simulink model "ECCE_tutorial_demo2_part1"  (R2022a)
settings: Solver=FixedStepAuto  StartTime=0.0  StopTime=10/60  FixedStep=1/12000  RelTol=1e-3
undefined symbols (not defined in the file or in its folder): Fault_Inv, GA_th_2, Vdc1, Vdc2, Vdc3, Vdc4, Vdc5
libraries: spsDCVoltageSourceLib x5, spsFullBridgeConverterLib x5, simulink x1, spsSeriesRLCBranchLib x1, spsAlphaBetaZerotodq0Lib x1, spsMeanLib x1, spsVoltageMeasurementLib x1, spspowerguiLib x1
settings Model: Creator=pgm  LastModifiedBy=pgm
settings DataIOCC: ReturnWorkspaceOutputs=off

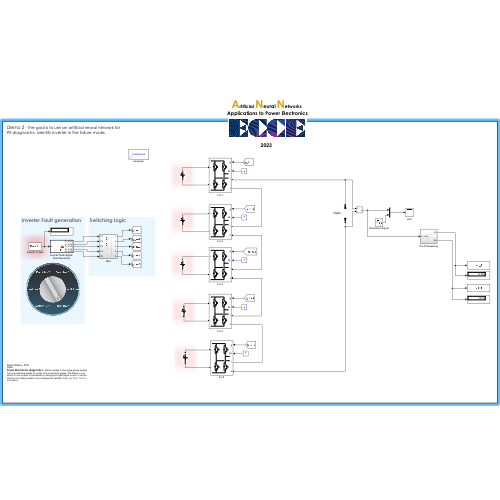
[thumbnail: Simulink's stored preview of the top-level diagram]
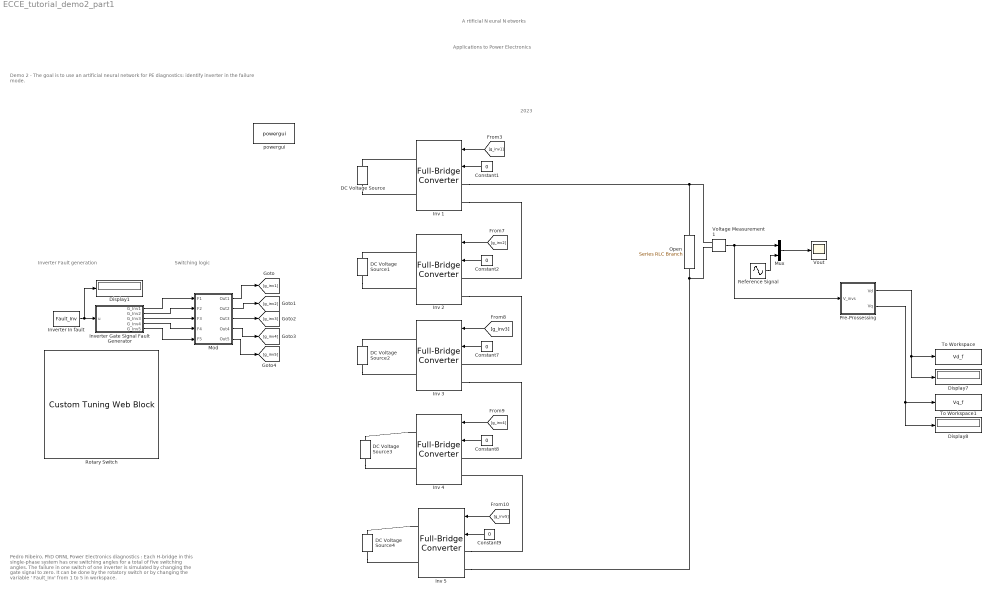
== system ECCE_tutorial_demo2_part1 ==
  note: A rtificial N eural N etworks
  note: Pedro Ribeiro, PhD
      | ORNL
      | Power Electronics diagnostics : Each H-bridge in this single-phase system has one switching angles for a total of five switching angles. The failure in one switch of one inverter is simulated by changing the gate signal to zero. It can be done by the rotatory switch or by changing the variable ' Fault_Inv' from 1 to 5 in workspace.
  note: Applications to Power Electronics
  note: 2023
  note: Demo 2 - The goal is to use an artificial neural network for PE diagnostics: identify inverter in the failure mode.
  note: Switching logic
  note: Inverter Fault generation
  Constant{1..2,7..9} (5 alike) : Constant  Value=0
  DC Voltage Source : spsDCVoltageSourceLib/DC Voltage Source  Amplitude=Vdc1  Measurements=None
  DC Voltage Source1 : spsDCVoltageSourceLib/DC Voltage Source  Amplitude=Vdc2  Measurements=None
  DC Voltage Source2 : spsDCVoltageSourceLib/DC Voltage Source  Amplitude=Vdc3  Measurements=None
  DC Voltage Source3 : spsDCVoltageSourceLib/DC Voltage Source  Amplitude=Vdc4  Measurements=None
  DC Voltage Source4 : spsDCVoltageSourceLib/DC Voltage Source  Amplitude=Vdc5  Measurements=None
  Display1 : Display
  Display7 : Display
  Display8 : Display
  Inv {1..5} (5 alike) : spsFullBridgeConverterLib/Full-Bridge Converter  ModelType=Switching devices  Ron=1e-3  Rs=1e6  Cs=inf  Vforward=[0,0]  Ron_Diode=1e-3  Rs_Diode=1e6  Cs_Diode=inf  Vf_Diode=1e-3  Rs_CurrentSource=inf  Ron_ACsource=1e-3
      settings: SourceProductBaseCode=PS
  Inverter Gate Signal Fault Generator : MATLAB Function  TreatAsAtomicUnit=on
  Inverter In fault : Constant  Value=Fault_Inv
  Mod : Subsystem
  Mux : Mux  Inputs=2
  Open : spsSeriesRLCBranchLib/Series RLC Branch  LConnTagsString=__new0  RConnTagsString=__new0  BranchType=Open circuit  Resistance=50  Inductance=3e-3  SetiL0=off  InitialCurrent=0  Capacitance=400e-6  Setx0=off  InitialVoltage=0  Measurements=None
  Pre-Prossessing : Subsystem
  Reference Signal : Sin  Amplitude=120*sqrt(2)  Frequency=2*pi*60  SampleTime=0
  Rotary Switch : CustomTuningWebBlock  LabelPosition=Hide  ShowInitialText=on  Configuration="{\"components\":[{\"name\":\"RotarySwitchComponent\",\"settings\":{\"arcAngle\":300,\"arcAngleOffset\":120,\"handle\":{\"size\":[150,150],\"src\":\"data:image\\/svg+xml;base64,PHN2ZyBpZD0iTGF5ZXJfMSIgZGF0YS1uYW1lPSJMYXllciAxIiB4bWxucz0iaHR0cDovL3d3dy53My5vcmcvMjAwMC9zdmciIHhtbG5zOnhsaW5rPSJodHRwOi8vd3d3LnczLm9yZy8xOTk5L3hsaW5rIiB2aWV3Qm94PSIwIDAgMTIxIDEyMSI+PGRlZnM+PHN0eWxlPi5jbHMtMXtmaWxsOnVybCgjbGluZWFyLWdyYWRpZW50KTt9LmNscy0yLC5jbHMtM3tmaWxsOiNkMWQxZDE7fS5jbHMtM3tzdHJva2U6I2I3YjdiNztzdHJva2UtbWl0ZXJsaW1pdDoxMDtzdHJva2Utd2lkdGg6MC4yNXB4O30uY2xzLTR7ZmlsbDojZjMwMDAwO30uY2xzLTV7ZmlsbDojZjIxNzY3O308L3N0eWxlPjxsaW5lYXJHcmFkaWVudCBpZD0ibGluZWFyLWdyYWRpZW50IiB4MT0iNjAuNSIgeTE9IjEyMC41IiB4Mj0iNjAuNSIgeTI9IjAuNSIgZ3JhZGllbnRVbml0cz0idXNlclNwYWNlT25Vc2UiPjxzdG9wIG9mZnNldD0iMCIgc3RvcC1jb2xvcj0iI2QxZDFkMSIvPjxzdG9wIG9mZnNldD0iMC4xIiBzdG9wLWNvbG9yPSIjY2VjZWNlIi8+PHN0b3Agb2Zmc2V0PSIwLjE5IiBzdG9wLWNvbG9yPSIjYzNjM2MzIi8+PHN0b3Agb2Zmc2V0PSIwLjI4IiBzdG9wLWNvbG9yPSIjYjFiMWIxIi8+PHN0b3Agb2Zmc2V0PSIwLjM2IiBzdG9wLWNvbG9yPSIjOTg5ODk4Ii8+PHN0b3Agb2Zmc2V0PSIwLjQ0IiBzdG9wLWNvbG9yPSIjNzg3ODc4Ii8+PHN0b3Agb2Zmc2V0PSIwLjQ2IiBzdG9wLWNvbG9yPSIjNmI2YjZiIi8+PHN0b3Agb2Zmc2V0PSIwLjU0IiBzdG9wLWNvbG9yPSIjNmI2YjZiIi8+PHN0b3Agb2Zmc2V0PSIwLjU2IiBzdG9wLWNvbG9yPSIjNzY3Njc2Ii8+PHN0b3Agb2Zmc2V0PSIwLjY0IiBzdG9wLWNvbG9yPSIjOTc5Nzk3Ii8+PHN0b3Agb2Zmc2V0PSIwLjcyIiBzdG9wLWNvbG9yPSIjYjBiMGIwIi8+PHN0b3Agb2Zmc2V0PSIwLjgxIiBzdG9wLWNvbG9yPSIjYzNjM2MzIi8+PHN0b3Agb2Zmc2V0PSIwLjkiIHN0b3AtY29sb3I9IiNjZGNkY2QiLz48c3RvcCBvZmZzZXQ9IjEiIHN0b3AtY29sb3I9IiNkMWQxZDEiLz48L2xpbmVhckdyYWRpZW50PjwvZGVmcz48Y2lyY2xlIGNsYXNzPSJjbHMtMSIgY3g9IjYwLjUiIGN5PSI2MC41IiByPSI2MCIvPjxwYXRoIGNsYXNzPSJjbHMtMiIgZD0iTTYwLjUsMUE1OS41LDU5LjUsMCwxLDEsMSw2MC41LDU5LjU3LDU5LjU3LDAsMCwxLDYwLjUsMW0wLTFBNjAuNSw2MC41LDAsMSwwLDEyMSw2MC41LDYwLjUsNjAuNSwwLDAsMCw2MC41LDBaIi8+PHJlY3QgY2xhc3M9ImNscy0zIiB4PSIwLjUiIHk9IjUxLjUiIHdpZHRoPSIxMjAiIGhlaWdodD0iMTgiIHJ4PSIzLjA0Ii8+PHJlY3QgY2xhc3M9ImNscy00IiB4PSI1Ljc1IiB5PSI1OC43NSIgd2lkdGg9IjE2IiBoZWlnaHQ9IjMiLz48cGF0aCBjbGFzcz0iY2xzLTUiIGQ9Ik0yMS4yNSw1OS4yNXYyaC0xNXYtMmgxNW0xLTFoLTE3djRoMTd2LTRaIi8+PC9zdmc+\"},\"handleOffset\":[0.00839802927552135,0],\"handleOrientation\":180,\"handlePosition\":[0,0,1,1],\"handleSize\":{\"height\":0.5,\"width\":0.5},\"labelRadius\":0.36,\"position\":[0,0,1,1],\"states\":[{\"Label\":{\"color\":[0,0,0,1],\"icon\":{\"size\":[0,0],\"src\":[],\"srcOrientation\":\"Right\"},\"iconPlacement\":\"left\",\"opacity\":1,\"position\":[0.7345552884615385,0.6796274038461538],\"show\":true,\"text\":{\"content\":\"Normal Op.\",\"font\":\"Helvetica\",\"fontSize\":24}},\"Value\":0},{\"Label\":{\"color\":[0,0,0,1],\"icon\":{\"size\":[0,0],\"src\":[],\"srcOrientation\":\"Right\"},\"iconPlacement\":\"left\",\"opacity\":1,\"position\":[0.35757211538461536,0.7603966346153846],\"show\":true,\"text\":{\"content\":\"Fault Inv1\",\"font\":\"Helvetica\",\"fontSize\":24}},\"Value\":1},{\"Label\":{\"color\":[0,0,0,1],\"icon\":{\"size\":[0,0],\"src\":[],\"srcOrientation\":\"Right\"},\"iconPlacement\":\"left\",\"opacity\":1,\"position\":[0.09603365384615385,0.46033653846153844],\"show\":true,\"text\":{\"content\":\"Fault Inv2\",\"font\":\"Helvetica\",\"fontSize\":24}},\"Value\":2},{\"Label\":{\"color\":[0,0,0,1],\"icon\":{\"size\":[0,0],\"src\":[],\"srcOrientation\":\"Right\"},\"iconPlacement\":\"left\",\"opacity\":1,\"position\":[0.36532451923076925,0.1180889423076923],\"show\":true,\"text\":{\"content\":\"Fault Inv3\",\"font\":\"Helvetica\",\"fontSize\":24}},\"Value\":3},{\"Label\":{\"color\":[0,0,0,1],\"icon\":{\"size\":[0,0],\"src\":[],\"srcOrientation\":\"Right\"},\"iconPlacement\":\"left\",\"opacity\":1,\"position\":[0.7191706730769231,0.19501201923076922],\"show\":true,\"text\":{\"content\":\"Fault Inv4\",\"font\":\"Helvetica\",\"fontSize\":24}},\"Value\":4},{\"Label\":{\"color\":[0,0,0],\"icon\":{\"size\":[1,1],\"src\":\"default\",\"srcOrientation\":\"Right\"},\"iconPlacement\":\"left\",\"opacity\":1,\"position\":[0,0],\"show\":true,\"text\":{\"content\":\"Fault Inv5\",\"fontSize\":14}},\"Value\":5}],\"tickRadius\":0.32}},{\"name\":\"BackgroundImageComponent\",\"settings\":{\"image\":{\"size\":[155,150],\"src\":\"data:image\\/svg+xml;base64,PD94bWwgdmVyc2lvbj0iMS4wIiBlbmNvZGluZz0idXRmLTgiPz4NCjwhLS0gR2VuZXJhdG9yOiBBZG9iZSBJbGx1c3RyYXRvciAyNS4wLjAsIFNWRyBFeHBvcnQgUGx1Zy1JbiAuIFNWRyBWZXJzaW9uOiA2LjAwIEJ1aWxkIDApICAtLT4NCjxzdmcgdmVyc2lvbj0iMS4xIg0KCSBpZD0iTGF5ZXJfMl8xXyIgeG1sbnM6Y2M9Imh0dHA6Ly9jcmVhdGl2ZWNvbW1vbnMub3JnL25zIyIgeG1sbnM6ZGM9Imh0dHA6Ly9wdXJsLm9yZy9kYy9lbGVtZW50cy8xLjEvIiB4bWxuczppbmtzY2FwZT0iaHR0cDovL3d3dy5pbmtzY2FwZS5vcmcv ...(+4184 chars)\",\"srcOrientation\":\"Right\"},\"position\":[0,0,1,1],\"scaleMode\":\"0\"}},{\"name\":\"ForegroundImageComponent\",\"settings\":{\"image\":{\"size\":[0,0],\"src\":\"default\",\"srcOrientation\":[]},\"isForeground\":1,\"position\":[0,0,1,1],\"scaleMode\":\"0\"}}],\"settings\":{\"BindingType\":\"param\",\"backgroundColor\":[0,0,255,\"1\"],\"enumDataType\":\"\",\"fixedAspectRatio\":\"on\",\"image\":{\"size\":[150,150],\"src\":\"data:image\\/svg+xml;base64,PD94bWwgdmVyc2lvbj0iMS4wIiBlbmNvZGluZz0iVVRGLTgiIHN0YW5kYWxvbmU9Im5vIj8+CjwhLS0gR2VuZXJhdG9yOiBBZG9iZSBJbGx1c3RyYXRvciAxOS4yLjEsIFNWRyBFeHBvcnQgUGx1Zy1JbiAuIFNWRyBWZXJzaW9uOiA2LjAwIEJ1aWxkIDApICAtLT4KCjxzdmcKICAgeG1sbnM6ZGM9Imh0dHA6Ly9wdXJsLm9yZy9kYy9lbGVtZW50cy8xLjEvIgogICB4bWxuczpjYz0iaHR0cDovL2NyZWF0aXZlY29tbW9ucy5vcmcvbnMjIgogICB4bWxuczpyZGY9Imh0dHA6Ly93d3cudzMub3JnLzE5OTkvMDIvMjItcmRmLXN5bnRh ...(+9660 chars)\"},\"showBackgroundColor\":false,\"useEnumDataType\":false,\"variant\":\"rotarySwitch\"},\"type\":\"RotarySwitch\"}"
  To Workspace : ToWorkspace  VariableName=Vd_f  SampleTime=-1
      settings: MaxDataPoints=1
  To Workspace1 : ToWorkspace  VariableName=Vq_f  SampleTime=-1
      settings: MaxDataPoints=1
  Voltage Measurement1 : spsVoltageMeasurementLib/Voltage Measurement  Tag=PoWeRsYsTeMmEaSuReMeNt  PhasorSimulation=off  OutputType=Magnitude  PSBequivalent=0
  Vout : Scope
  powergui : spspowerguiLib/powergui  Priority=1  SimulationMode=Continuous  SampleTime=1e-6  frequency=60  Iterations=50  frequencyindice=0  Pbase=100e6  ErrMax=1e-4  UnitsV=kV  UnitsW=MW  buscounter=0  FunctionMessages=off  echomessages=off  EnableUseOfTLC=off  CurrentSourceSwitches=off  DisableSnubberDevices=off  DisableRonSwitches=off  DisableVfSwitches=off  DisplayEquations=off  AutomaticDiscreteSolvers=off  SolverType=Tustin/Backward Euler (TBE)  Interpol=off  ExternalGateDelay=off  methode=off  Ts=100  x0status=blocks  SPID=on  SwTol=0  HookPort=off  NonlinearTolerance=1e-4  nMaxIteration=100  ContinueOnMaxIteration=off  RestoreLinks=warning  ResistiveCurrentMeasurement=off  Frange=[0:2:500]  Ylog=off  Xlog=on  ShowGrid=off  save=off  variable=ZData  structure=0  ZoomFFT=off  StartTime=0.0  cycles=1  DisplayStyle=1  fundamental=60  FreqAxis=off  MaxFrequency=1000  frequencyindicesteady=1  RmsSteady=1  display=off
  wires:
  Constant1/1 -> Inv 1/2
  Constant2/1 -> Inv 2/2
  [g_inv1] -> Inv 1/1
  [g_inv2] -> Inv 2/1
  [g_inv4] -> Inv 4/1
  [g_inv3] -> Inv 3/1
  Constant8/1 -> Inv 4/2
  Constant7/1 -> Inv 3/2
  Constant9/1 -> Inv 5/2
  [g_inv5] -> Inv 5/1
  Reference Signal/1 -> Mux/2
  Mux/1 -> Vout/1
  Voltage Measurement1/1 -> Mux/1, Pre-Prossessing/1(V_invs)
  Inverter Gate Signal Fault Generator/1(G_Inv1) -> Mod/1(F1)
  Inverter Gate Signal Fault Generator/2(G_Inv2) -> Mod/2(F2)
  Inverter Gate Signal Fault Generator/3(G_Inv3) -> Mod/3(F3)
  Inverter Gate Signal Fault Generator/4(G_Inv4) -> Mod/4(F4)
  Inverter Gate Signal Fault Generator/5(G_Inv5) -> Mod/5(F5)
  Mod/1(Out1) -> [g_inv1]
  Mod/2(Out2) -> [g_inv2]
  Mod/3(Out3) -> [g_inv3]
  Mod/4(Out4) -> [g_inv4]
  Mod/5(Out5) -> [g_inv5]
  Pre-Prossessing/1(Vd) -> Display7/1, To Workspace/1
  Pre-Prossessing/2(Vq) -> Display8/1, To Workspace1/1
  Inverter In fault/1 -> Display1/1, Inverter Gate Signal Fault Generator/1(u)
  connections:
  DC Voltage Source/RConn1 -- Inv 1/RConn1
  DC Voltage Source/LConn1 -- Inv 1/RConn2
  Inv 2/RConn1 -- DC Voltage Source1/RConn1
  DC Voltage Source1/LConn1 -- Inv 2/RConn2
  Voltage Measurement1/LConn2 -- Inv 5/LConn2 -- Open/RConn1
  Voltage Measurement1/LConn1 -- Inv 1/LConn1 -- Open/LConn1
  Inv 4/RConn1 -- DC Voltage Source3/RConn1
  DC Voltage Source2/LConn1 -- Inv 3/RConn2
  DC Voltage Source3/LConn1 -- Inv 4/RConn2
  DC Voltage Source2/RConn1 -- Inv 3/RConn1
  DC Voltage Source4/LConn1 -- Inv 5/RConn2
  Inv 5/RConn1 -- DC Voltage Source4/RConn1
  Inv 1/LConn2 -- Inv 2/LConn1
  Inv 2/LConn2 -- Inv 3/LConn1
  Inv 3/LConn2 -- Inv 4/LConn1
  Inv 5/LConn1 -- Inv 4/LConn2

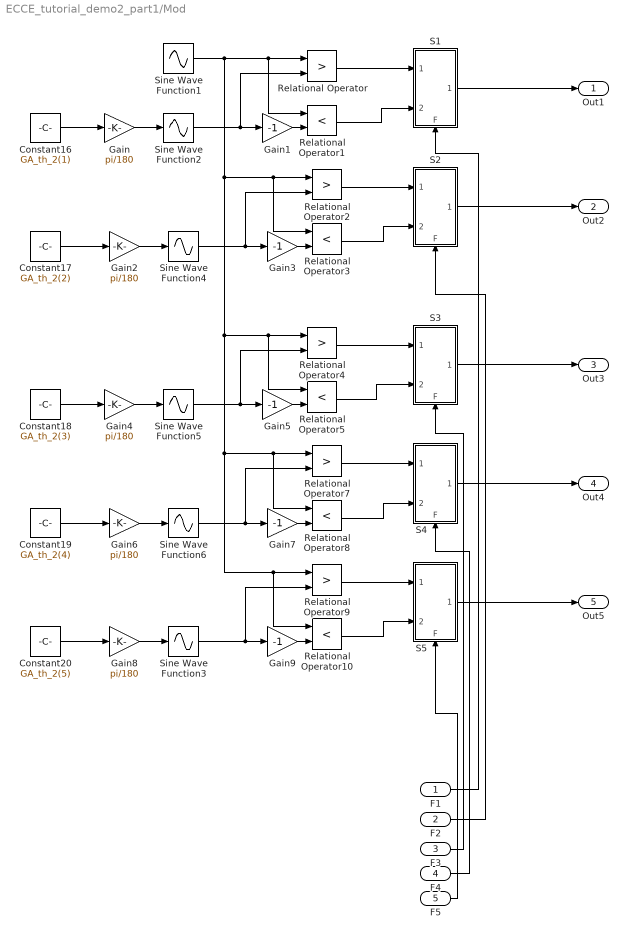
== system ECCE_tutorial_demo2_part1/Mod ==
  F1 : Inport
  F2 : Inport  Port=2
  F3 : Inport  Port=3
  F4 : Inport  Port=4
  F5 : Inport  Port=5
  Constant16 : Constant  Value=GA_th_2(1)
  Constant17 : Constant  Value=GA_th_2(2)
  Constant18 : Constant  Value=GA_th_2(3)
  Constant19 : Constant  Value=GA_th_2(4)
  Constant20 : Constant  Value=GA_th_2(5)
  Gain{,2,4,6,8} (5 alike) : Gain  Gain=pi/180
  Gain{1,3,5,7,9} (5 alike) : Gain  Gain=-1
  Relational Operator{,2,4,7,9} (5 alike) : RelationalOperator  Operator=>  OutDataTypeStr=boolean  RndMeth=Simplest  InputSameDT=off
  Relational Operator{1,3,5,8,10} (5 alike) : RelationalOperator  Operator=<  OutDataTypeStr=boolean  RndMeth=Simplest  InputSameDT=off
  S1 : Subsystem
      settings: PortSchema="{\"entries\":[{\"content\":{\"sides\":[{\"content\":{\"connectorIds\":[\"In1\",\"In2\"]},\"type\":\"ConnectorPlacement.EquallySpacedRectSide\",\"uuid\":\"5f14345d-2d5d-483d-90d8-8aa8f8d7da25\"},{\"content\":{\"connectorIds\":[\"Out1\"],\"side\":\"RIGHT\"},\"type\":\"ConnectorPlacement.EquallySpacedRectSide\",\"uuid\":\"3e161696-ca31-43e2-b7bf-a13ac7fb6ba1\"},{\"content\":{\"connectorIds\":[],\"side\":\"TOP\"},\"type\":\"ConnectorPlacement.EquallySpacedRectSide\",\"uuid\":\"8fa02895-2f1e-47bd-8a65-8e37c65d1a87\"},{\"content\":{\"connectorIds\":[\"In3\"],\"side\":\"BOTTOM\"},\"type\":\"ConnectorPlacement.EquallySpacedRectSide\",\"uuid\":\"36cd283d-056f-45a3-b6f0-6bf0daee5395\"}]},\"type\":\"ConnectorPlacement.EquallySpacedConnector\",\"uuid\":\"d0616103-6a76-4dfd-bdc2-221e478031b1\"}],\"packageUris\":[\"http://schema.mathworks.com/mf0/Connector/R2020b\"],\"version\":\"1.0\"}"
  S2 : Subsystem
      settings: PortSchema="{\"entries\":[{\"content\":{\"sides\":[{\"content\":{\"connectorIds\":[\"In1\",\"In2\"]},\"type\":\"ConnectorPlacement.EquallySpacedRectSide\",\"uuid\":\"5f14345d-2d5d-483d-90d8-8aa8f8d7da25\"},{\"content\":{\"connectorIds\":[\"Out1\"],\"side\":\"RIGHT\"},\"type\":\"ConnectorPlacement.EquallySpacedRectSide\",\"uuid\":\"3e161696-ca31-43e2-b7bf-a13ac7fb6ba1\"},{\"content\":{\"connectorIds\":[],\"side\":\"TOP\"},\"type\":\"ConnectorPlacement.EquallySpacedRectSide\",\"uuid\":\"8fa02895-2f1e-47bd-8a65-8e37c65d1a87\"},{\"content\":{\"connectorIds\":[\"In3\"],\"side\":\"BOTTOM\"},\"type\":\"ConnectorPlacement.EquallySpacedRectSide\",\"uuid\":\"712a4502-34e9-4038-bdd0-4ff6e3ff4ab9\"}]},\"type\":\"ConnectorPlacement.EquallySpacedConnector\",\"uuid\":\"d0616103-6a76-4dfd-bdc2-221e478031b1\"}],\"packageUris\":[\"http://schema.mathworks.com/mf0/Connector/R2020b\"],\"version\":\"1.0\"}"
  S3 : Subsystem
      settings: PortSchema="{\"entries\":[{\"content\":{\"sides\":[{\"content\":{\"connectorIds\":[\"In1\",\"In2\"]},\"type\":\"ConnectorPlacement.EquallySpacedRectSide\",\"uuid\":\"5f14345d-2d5d-483d-90d8-8aa8f8d7da25\"},{\"content\":{\"connectorIds\":[\"Out1\"],\"side\":\"RIGHT\"},\"type\":\"ConnectorPlacement.EquallySpacedRectSide\",\"uuid\":\"3e161696-ca31-43e2-b7bf-a13ac7fb6ba1\"},{\"content\":{\"connectorIds\":[],\"side\":\"TOP\"},\"type\":\"ConnectorPlacement.EquallySpacedRectSide\",\"uuid\":\"8fa02895-2f1e-47bd-8a65-8e37c65d1a87\"},{\"content\":{\"connectorIds\":[\"In3\"],\"side\":\"BOTTOM\"},\"type\":\"ConnectorPlacement.EquallySpacedRectSide\",\"uuid\":\"dcf360f9-50cf-4544-a649-25291c772c87\"}]},\"type\":\"ConnectorPlacement.EquallySpacedConnector\",\"uuid\":\"d0616103-6a76-4dfd-bdc2-221e478031b1\"}],\"packageUris\":[\"http://schema.mathworks.com/mf0/Connector/R2020b\"],\"version\":\"1.0\"}"
  S4 : Subsystem
      settings: PortSchema="{\"entries\":[{\"content\":{\"sides\":[{\"content\":{\"connectorIds\":[\"In1\",\"In2\"]},\"type\":\"ConnectorPlacement.EquallySpacedRectSide\",\"uuid\":\"5f14345d-2d5d-483d-90d8-8aa8f8d7da25\"},{\"content\":{\"connectorIds\":[\"Out1\"],\"side\":\"RIGHT\"},\"type\":\"ConnectorPlacement.EquallySpacedRectSide\",\"uuid\":\"3e161696-ca31-43e2-b7bf-a13ac7fb6ba1\"},{\"content\":{\"connectorIds\":[],\"side\":\"TOP\"},\"type\":\"ConnectorPlacement.EquallySpacedRectSide\",\"uuid\":\"8fa02895-2f1e-47bd-8a65-8e37c65d1a87\"},{\"content\":{\"connectorIds\":[\"In3\"],\"side\":\"BOTTOM\"},\"type\":\"ConnectorPlacement.EquallySpacedRectSide\",\"uuid\":\"86d75a55-3df2-435d-b886-235f200f3608\"}]},\"type\":\"ConnectorPlacement.EquallySpacedConnector\",\"uuid\":\"d0616103-6a76-4dfd-bdc2-221e478031b1\"}],\"packageUris\":[\"http://schema.mathworks.com/mf0/Connector/R2020b\"],\"version\":\"1.0\"}"
  S5 : Subsystem
      settings: PortSchema="{\"entries\":[{\"content\":{\"sides\":[{\"content\":{\"connectorIds\":[\"In1\",\"In2\"]},\"type\":\"ConnectorPlacement.EquallySpacedRectSide\",\"uuid\":\"5f14345d-2d5d-483d-90d8-8aa8f8d7da25\"},{\"content\":{\"connectorIds\":[\"Out1\"],\"side\":\"RIGHT\"},\"type\":\"ConnectorPlacement.EquallySpacedRectSide\",\"uuid\":\"3e161696-ca31-43e2-b7bf-a13ac7fb6ba1\"},{\"content\":{\"connectorIds\":[],\"side\":\"TOP\"},\"type\":\"ConnectorPlacement.EquallySpacedRectSide\",\"uuid\":\"8fa02895-2f1e-47bd-8a65-8e37c65d1a87\"},{\"content\":{\"connectorIds\":[\"In3\"],\"side\":\"BOTTOM\"},\"type\":\"ConnectorPlacement.EquallySpacedRectSide\",\"uuid\":\"319f308e-a951-488d-98cf-79dcc4f9ddf4\"}]},\"type\":\"ConnectorPlacement.EquallySpacedConnector\",\"uuid\":\"d0616103-6a76-4dfd-bdc2-221e478031b1\"}],\"packageUris\":[\"http://schema.mathworks.com/mf0/Connector/R2020b\"],\"version\":\"1.0\"}"
  Sine Wave Function1 : Sin  Frequency=2*pi*60  SampleTime=0
  Sine Wave Function{2..6} (5 alike) : Sin  TimeSource=Use external signal  SampleTime=0
  Out1 : Outport
  Out2 : Outport  Port=2
  Out3 : Outport  Port=3
  Out4 : Outport  Port=4
  Out5 : Outport  Port=5
  wires:
  Gain5/1 -> Relational Operator5/2
  Relational Operator10/1 -> S5/2(In1)
  Relational Operator4/1 -> S3/1(In2)
  Sine Wave Function2/1 -> Gain1/1, Relational Operator/2
  Sine Wave Function3/1 -> Relational Operator9/2, Gain9/1
  Gain4/1 -> Sine Wave Function5/1
  Relational Operator/1 -> S1/1(In2)
  Sine Wave Function4/1 -> Relational Operator2/2, Gain3/1
  Relational Operator9/1 -> S5/1(In2)
  Gain9/1 -> Relational Operator10/2
  S5/1(Out1) -> Out5/1
  Gain/1 -> Sine Wave Function2/1
  Sine Wave Function1/1 -> Relational Operator4/1, Relational Operator5/1, Relational Operator9/1, Relational Operator10/1, Relational Operator8/1, Relational Operator7/1, Relational Operator2/1, Relational Operator3/1, Relational Operator1/1, Relational Operator/1
  Gain7/1 -> Relational Operator8/2
  Gain6/1 -> Sine Wave Function6/1
  Sine Wave Function6/1 -> Gain7/1, Relational Operator7/2
  Sine Wave Function5/1 -> Relational Operator4/2, Gain5/1
  S2/1(Out1) -> Out2/1
  Relational Operator3/1 -> S2/2(In1)
  Constant20/1 -> Gain8/1
  S3/1(Out1) -> Out3/1
  F2/1 -> S2/3(F)
  F1/1 -> S1/3(F)
  Relational Operator2/1 -> S2/1(In2)
  Relational Operator1/1 -> S1/2(In1)
  Constant17/1 -> Gain2/1
  Constant16/1 -> Gain/1
  Gain3/1 -> Relational Operator3/2
  Relational Operator8/1 -> S4/2(In1)
  Gain1/1 -> Relational Operator1/2
  Gain2/1 -> Sine Wave Function4/1
  Constant19/1 -> Gain6/1
  Relational Operator7/1 -> S4/1(In2)
  Constant18/1 -> Gain4/1
  Relational Operator5/1 -> S3/2(In1)
  Gain8/1 -> Sine Wave Function3/1
  S1/1(Out1) -> Out1/1
  S4/1(Out1) -> Out4/1
  F4/1 -> S4/3(F)
  F5/1 -> S5/3(F)
  F3/1 -> S3/3(F)

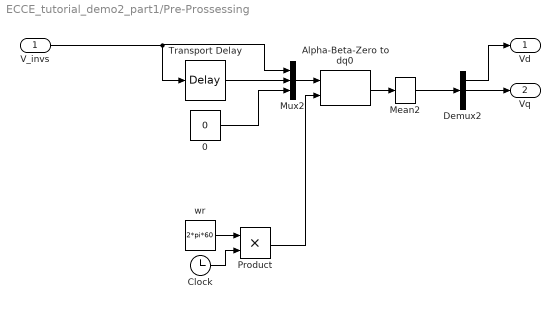
== system ECCE_tutorial_demo2_part1/Pre-Prossessing ==
  V_invs : Inport
  0 : Constant  Value=0
  Alpha-Beta-Zero to dq0 : spsAlphaBetaZerotodq0Lib/Alpha-Beta-Zero to dq0  Alignment=Aligned with phase A axis
      settings: SourceProductBaseCode=PS
  Clock : Clock
  Demux2 : Demux  Outputs=3
  Mean2 : spsMeanLib/Mean  Freq=60  Vinit=0  Ts=0
  Mux2 : Mux  Inputs=3
  Product : Product
  Transport Delay : TransportDelay  DelayTime=(1/60)/4
  wr : Constant  Value=2*pi*60
  Vd : Outport
  Vq : Outport  Port=2
  wires:
  Mux2/1 -> Alpha-Beta-Zero to dq0/1
  Mean2/1 -> Demux2/1
  Demux2/2 -> Vq/1
  Product/1 -> Alpha-Beta-Zero to dq0/2
  Transport Delay/1 -> Mux2/2
  wr/1 -> Product/1
  Clock/1 -> Product/2
  0/1 -> Mux2/3
  Alpha-Beta-Zero to dq0/1 -> Mean2/1
  V_invs/1 -> Mux2/1, Transport Delay/1
  Demux2/1 -> Vd/1

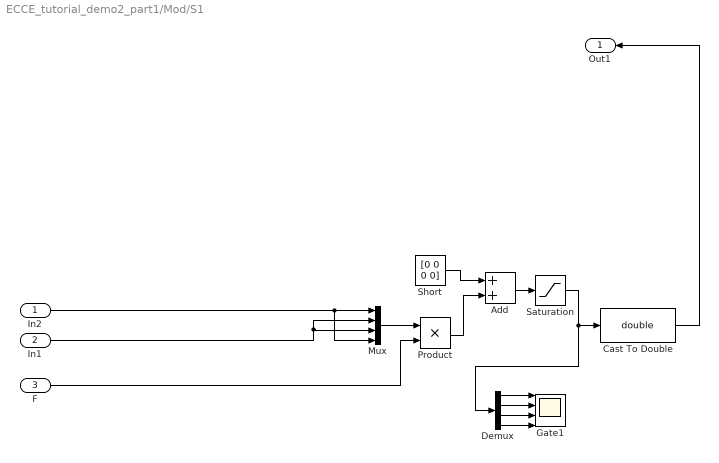
== system ECCE_tutorial_demo2_part1/Mod/S1 ==
  In2 : Inport
  In1 : Inport  Port=2
  F : Inport  Port=3
  Add : Sum
  Cast To Double : DataTypeConversion  OutDataTypeStr=double  SaturateOnIntegerOverflow=off  RndMeth=Floor
  Demux : Demux
  Gate1 : Scope  NumInputPorts=4
  Mux : Mux
  Product : Product
  Saturation : Saturate  UpperLimit=1  LowerLimit=0
  Short : Constant  Value=[0 0 0 0]
  Out1 : Outport
  wires:
  Mux/1 -> Product/1
  Cast To Double/1 -> Out1/1
  In2/1 -> Mux/4, Mux/1
  In1/1 -> Mux/3, Mux/2
  Product/1 -> Add/2
  Demux/1 -> Gate1/1
  Demux/2 -> Gate1/2
  Demux/3 -> Gate1/3
  Demux/4 -> Gate1/4
  Short/1 -> Add/1
  Add/1 -> Saturation/1
  Saturation/1 -> Demux/1, Cast To Double/1
  F/1 -> Product/2

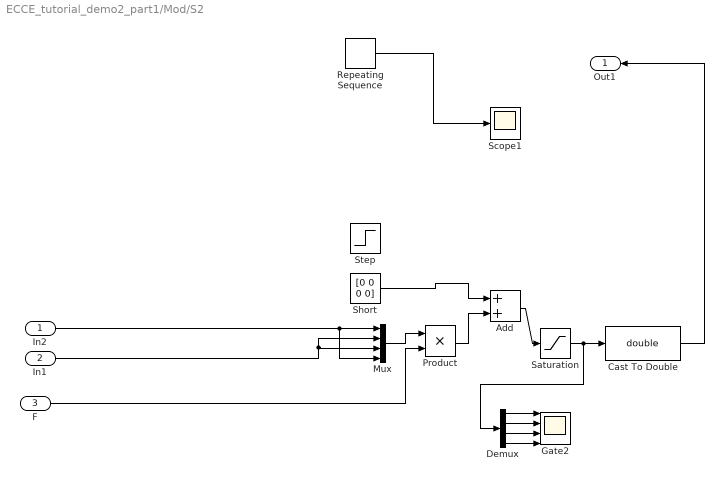
== system ECCE_tutorial_demo2_part1/Mod/S2 ==
  In2 : Inport
  In1 : Inport  Port=2
  F : Inport  Port=3
  Add : Sum
  Cast To Double : DataTypeConversion  OutDataTypeStr=double  SaturateOnIntegerOverflow=off  RndMeth=Floor
  Demux : Demux
  Gate2 : Scope  NumInputPorts=4
  Mux : Mux
  Product : Product
  Repeating Sequence : simulink/Sources/Repeating Sequence  rep_seq_t="[0  3/60 3.01/60 20/60 20.01/60 30/60 ]"  rep_seq_y="[1 1  1 1 1 1 ]"
  Saturation : Saturate  UpperLimit=1  LowerLimit=0
  Scope1 : Scope
  Short : Constant  Value=[0 0 0 0]
  Step : Step  Time=10/60  SampleTime=0
  Out1 : Outport
  wires:
  Repeating Sequence/1 -> Scope1/1
  Short/1 -> Add/1
  Saturation/1 -> Cast To Double/1, Demux/1
  Add/1 -> Saturation/1
  Demux/4 -> Gate2/4
  Demux/3 -> Gate2/3
  Demux/2 -> Gate2/2
  Demux/1 -> Gate2/1
  Product/1 -> Add/2
  In1/1 -> Mux/2, Mux/3
  In2/1 -> Mux/1, Mux/4
  Cast To Double/1 -> Out1/1
  Mux/1 -> Product/1
  F/1 -> Product/2

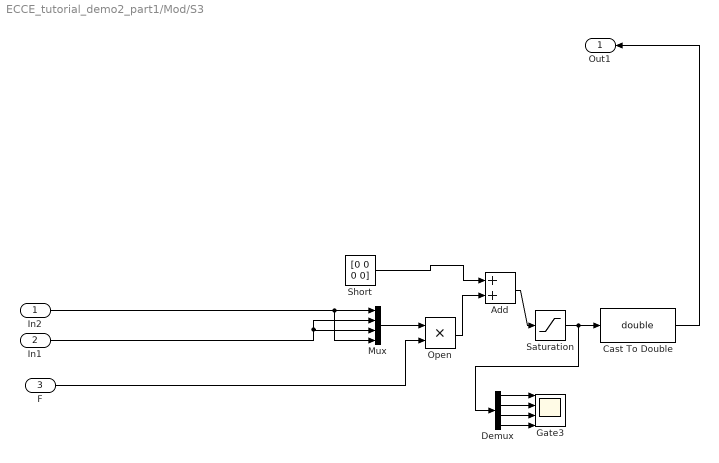
== system ECCE_tutorial_demo2_part1/Mod/S3 ==
  In2 : Inport
  In1 : Inport  Port=2
  F : Inport  Port=3
  Add : Sum
  Cast To Double : DataTypeConversion  OutDataTypeStr=double  SaturateOnIntegerOverflow=off  RndMeth=Floor
  Demux : Demux
  Gate3 : Scope  NumInputPorts=4
  Mux : Mux
  Open : Product
  Saturation : Saturate  UpperLimit=1  LowerLimit=0
  Short : Constant  Value=[0 0 0 0]
  Out1 : Outport
  wires:
  Mux/1 -> Open/1
  Cast To Double/1 -> Out1/1
  In2/1 -> Mux/4, Mux/1
  In1/1 -> Mux/3, Mux/2
  Open/1 -> Add/2
  Demux/1 -> Gate3/1
  Demux/2 -> Gate3/2
  Demux/3 -> Gate3/3
  Demux/4 -> Gate3/4
  Add/1 -> Saturation/1
  Saturation/1 -> Demux/1, Cast To Double/1
  Short/1 -> Add/1
  F/1 -> Open/2

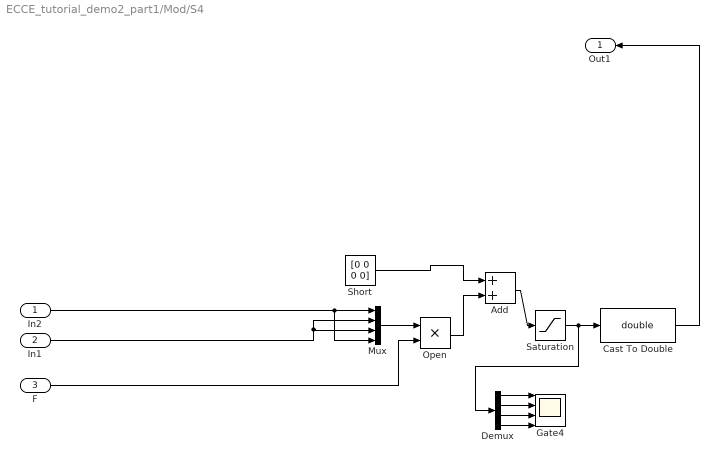
== system ECCE_tutorial_demo2_part1/Mod/S4 ==
  In2 : Inport
  In1 : Inport  Port=2
  F : Inport  Port=3
  Add : Sum
  Cast To Double : DataTypeConversion  OutDataTypeStr=double  SaturateOnIntegerOverflow=off  RndMeth=Floor
  Demux : Demux
  Gate4 : Scope  NumInputPorts=4
  Mux : Mux
  Open : Product
  Saturation : Saturate  UpperLimit=1  LowerLimit=0
  Short : Constant  Value=[0 0 0 0]
  Out1 : Outport
  wires:
  Short/1 -> Add/1
  Saturation/1 -> Cast To Double/1, Demux/1
  Add/1 -> Saturation/1
  Demux/4 -> Gate4/4
  Demux/3 -> Gate4/3
  Demux/2 -> Gate4/2
  Demux/1 -> Gate4/1
  Open/1 -> Add/2
  In1/1 -> Mux/2, Mux/3
  In2/1 -> Mux/1, Mux/4
  Cast To Double/1 -> Out1/1
  Mux/1 -> Open/1
  F/1 -> Open/2

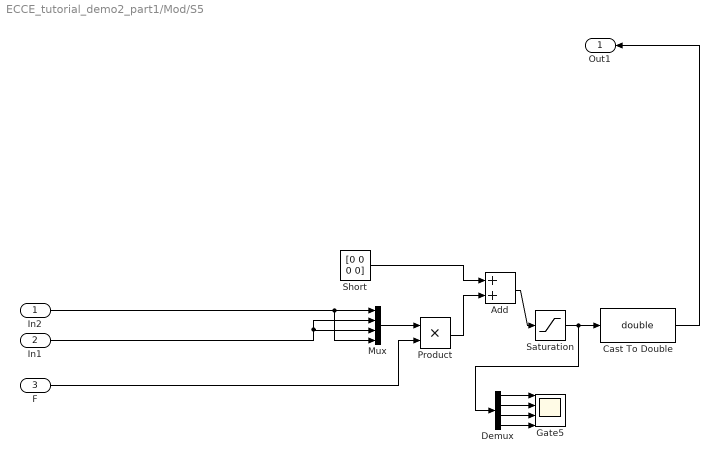
== system ECCE_tutorial_demo2_part1/Mod/S5 ==
  In2 : Inport
  In1 : Inport  Port=2
  F : Inport  Port=3
  Add : Sum
  Cast To Double : DataTypeConversion  OutDataTypeStr=double  SaturateOnIntegerOverflow=off  RndMeth=Floor
  Demux : Demux
  Gate5 : Scope  NumInputPorts=4
  Mux : Mux
  Product : Product
  Saturation : Saturate  UpperLimit=1  LowerLimit=0
  Short : Constant  Value=[0 0 0 0]
  Out1 : Outport
  wires:
  Mux/1 -> Product/1
  Cast To Double/1 -> Out1/1
  In2/1 -> Mux/4, Mux/1
  In1/1 -> Mux/3, Mux/2
  Product/1 -> Add/2
  Demux/1 -> Gate5/1
  Demux/2 -> Gate5/2
  Demux/3 -> Gate5/3
  Demux/4 -> Gate5/4
  Add/1 -> Saturation/1
  Saturation/1 -> Demux/1, Cast To Double/1
  Short/1 -> Add/1
  F/1 -> Product/2

== matlab function ECCE_tutorial_demo2_part1/Inverter Gate Signal Fault Generator ==
  data: u input; G_Inv1 output; G_Inv2 output; G_Inv3 output; G_Inv4 output; G_Inv5 output
function [G_Inv1,G_Inv2,G_Inv3, G_Inv4,G_Inv5]= fcn(u)
%% Normal Operation
    G_Inv1 = [1 1 1 1]; 
    G_Inv2 = [1 1 1 1]; 
    G_Inv3 = [1 1 1 1]; 
    G_Inv4 = [1 1 1 1]; 
    G_Inv5 = [1 1 1 1]; 
if u==1 % Inv 1 Fault Operation
    G_Inv1 = [0 1 1 1]; 
    G_Inv2 = [1 1 1 1]; 
    G_Inv3 = [1 1 1 1]; 
    G_Inv4 = [1 1 1 1]; 
    G_Inv5 = [1 1 1 1]; 
end
if u==2 % Inv 2 Fault Operation
    G_Inv1 = [1 1 1 1]; 
    G_Inv2 = [1 0 1 1]; 
    G_Inv3 = [1 1 1 1]; 
    G_Inv4 = [1 1 1 1]; 
    G_Inv5 = [1 1 1 1]; 
end
if u==3 % Inv 3 Fault Operation
    G_Inv1 = [1 1 1 1]; 
    G_Inv2 = [1 1 1 1]; 
    G_Inv3 = [1 0 1 1]; 
    G_Inv4 = [1 1 1 1]; 
    G_Inv5 = [1 1 1 1]; 
end
if u==4 % Inv 4 Fault Operation
    G_Inv1 = [1 1 1 1]; 
    G_Inv2 = [1 1 1 1]; 
    G_Inv3 = [1 1 1 1]; 
    G_Inv4 = [1 1 0 1]; 
    G_Inv5 = [1 1 1 1]; 
end

if u==5 % Inv 5 Fault Operation
    G_Inv1 = [1 1 1 1]; 
    G_Inv2 = [1 1 1 1]; 
    G_Inv3 = [1 1 1 1]; 
    G_Inv4 = [1 1 1 1]; 
    G_Inv5 = [1 1 1 0]; 
end

end

% open_system('ECCE_tutorial_demo2_part1.slx'/Gate1')
